simulink model "box_model"  (R2018b)
settings: Solver=VariableStepAuto  StartTime=0.0  StopTime=10.0  RelTol=1e-3
values from neighbouring files (symbols this model uses):
  Aw1 = pi*r1^2    (= 0.000804247719319)    [gryf.m]
  g = 9.80665    [gryf.m]
  H1 = 1.9    [gryf.m]
undefined symbols (not defined in the file or in its folder): A1, h10
settings Model: Creator=gosci  LastModifiedBy=gosci

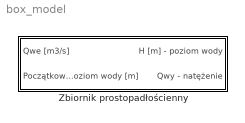
== system box_model ==
  Zbiornik prostopadłościenny : Subsystem

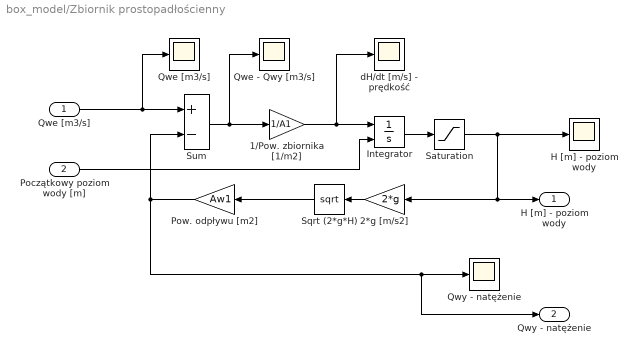
== system box_model/Zbiornik prostopadłościenny ==
  "Qwe [m3/s] " : Inport
  Początkowy poziom wody [m] : Inport  Port=2
  1/Pow. zbiornika [1/m2] : Gain  Gain=1/A1
  2*g [m/s2] : Gain  Gain=2*g
  H [m] - poziom wody : Scope
  Integrator : Integrator  InitialConditionSource=external  InitialCondition=h10
  Pow. odpływu [m2] : Gain  Gain=Aw1
  Qwe - Qwy [m3/s] : Scope
  Qwe [m3/s] : Scope
  Qwy - natężenie : Scope
  Saturation : Saturate  UpperLimit=H1  LowerLimit=0.01
  Sqrt (2*g*H) : Sqrt  SaturateOnIntegerOverflow=on
  Sum : Sum  Inputs=+-
  "dH/dt [m/s] - prędkość " : Scope
  "H [m] - poziom wody " : Outport
  "Qwy - natężenie " : Outport  Port=2
  wires:
  Sum/1 -> 1/Pow. zbiornika [1/m2]/1, Qwe - Qwy [m3/s]/1
  Saturation/1 -> H [m] - poziom wody/1, 2*g [m/s2]/1, "H [m] - poziom wody "/1
  Pow. odpływu [m2]/1 -> "Qwy - natężenie "/1, Qwy - natężenie/1, Sum/2
  Sqrt (2*g*H)/1 -> Pow. odpływu [m2]/1
  "Qwe [m3/s] "/1 -> Qwe [m3/s]/1, Sum/1
  1/Pow. zbiornika [1/m2]/1 -> Integrator/1, "dH/dt [m/s] - prędkość "/1
  2*g [m/s2]/1 -> Sqrt (2*g*H)/1
  Początkowy poziom wody [m]/1 -> Integrator/2
  Integrator/1 -> Saturation/1
